simulink model "Sum2"  (R2020b)
settings: Solver=VariableStepAuto  StartTime=0.0  StopTime=100  RelTol=1e-3
PreLoadFcn:
  | clc;
  | close all;
  | clear all;
  | m1=465;
  | m2=135;
  | k1=5700;
  | k2=135000;
  | b=290;
  | F=1;
settings Model: Creator=Aradhana desai  LastModifiedBy=Aradhana desai

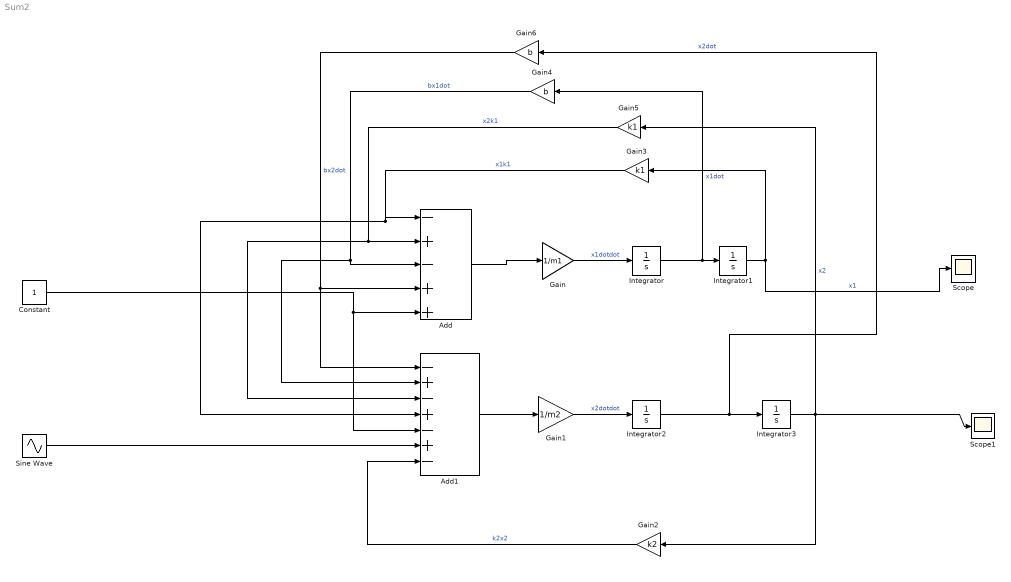
== system Sum2 ==
  Add : Sum  Inputs=-+-++
  Add1 : Sum  Inputs=-+-+-+-
  Constant : Constant
  Gain : Gain  Gain=1/m1
  Gain1 : Gain  Gain=1/m2
  Gain2 : Gain  Gain=k2
  Gain3 : Gain  Gain=k1
  Gain4 : Gain  Gain=b
  Gain5 : Gain  Gain=k1
  Gain6 : Gain  Gain=b
  Integrator{,1..3} (4 alike) : Integrator
  Scope : Scope
  Scope1 : Scope
  Sine Wave : Sin  Amplitude=k2  SampleTime=0
  wires:
  Add/1 -> Gain/1
  Gain/1 -> Integrator/1  "x1dotdot"
  Integrator/1 -> Gain4/1, Integrator1/1  "x1dot"
  Add1/1 -> Gain1/1
  Gain1/1 -> Integrator2/1  "x2dotdot"
  Integrator2/1 -> Integrator3/1, Gain6/1  "x2dot"
  Integrator3/1 -> Gain2/1, Scope1/1, Gain5/1  "x2"
  Integrator1/1 -> Gain3/1, Scope/1  "x1"
  Gain4/1 -> Add1/2, Add/3  "bx1dot"
  Gain3/1 -> Add1/4, Add/1  "x1k1"
  Gain5/1 -> Add1/3, Add/2  "x2k1"
  Gain6/1 -> Add1/1, Add/4  "bx2dot"
  Gain2/1 -> Add1/7  "k2x2"
  Constant/1 -> Add/5, Add1/5
  Sine Wave/1 -> Add1/6
